simulink model "Exercitiul3"  (R2016a)
settings: Solver=VariableStepDiscrete  StartTime=0.0  StopTime=10080  RelTol=1e-3
undefined symbols (not defined in the file): m, n
settings Model: Creator=Cristina  LastModifiedBy=Cristina

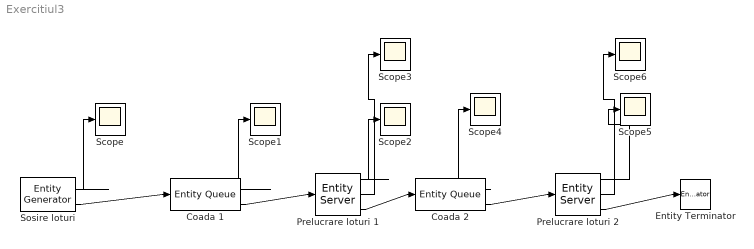
== system Exercitiul3 ==
  Coada 1 : EntityQueue  InputPortMessageModes=m  OutputPortMessageModes=n,m  Capacity=100  NumberEntitiesInBlock=on
      settings: OutputPortMap=o1,o5
  "Coada 2 " : EntityQueue  InputPortMessageModes=m  OutputPortMessageModes=n,m  Capacity=100  NumberEntitiesInBlock=on
      settings: OutputPortMap=o1,o5
  Entity Terminator : EntityTerminator  InputPortMessageModes=m
  Prelucrare loturi 1 : EntityServer  InputPortMessageModes=m  OutputPortMessageModes=n,n,m  Capacity=1  ServiceTimeValue=14  NumberEntitiesDeparted=on  Utilization=on
      settings: OutputPortMap=o0,o5,o9
  "Prelucrare loturi 2 " : EntityServer  InputPortMessageModes=m  OutputPortMessageModes=n,n,m  Capacity=1  ServiceTimeValue=3  NumberEntitiesDeparted=on  Utilization=on
      settings: OutputPortMap=o0,o5,o9
  Scope{,1..6} (7 alike) : Scope
  "Sosire loturi " : EntityGenerator  OutputPortMessageModes=n,m  TimeSource=MATLAB action  IntergenerationTimeAction=|  NumberEntitiesDeparted=on  EntityType=Structured  EntityTypeName=Entity
      | persistent init
      | if (isempty(init))
      |     rng(123);
      |     init = true;
      | end
      | dt = 12 + rand * 10;
      settings: OutputPortMap=o0,o3
  wires:
  "Sosire loturi "/2 -> Coada 1/1
  Coada 1/2 -> Prelucrare loturi 1/1
  Prelucrare loturi 1/3 -> "Coada 2 "/1
  "Coada 2 "/2 -> "Prelucrare loturi 2 "/1
  "Prelucrare loturi 2 "/3 -> Entity Terminator/1
  "Sosire loturi "/1 -> Scope/1
  Coada 1/1 -> Scope1/1
  Prelucrare loturi 1/1 -> Scope2/1
  Prelucrare loturi 1/2 -> Scope3/1
  "Coada 2 "/1 -> Scope4/1
  "Prelucrare loturi 2 "/1 -> Scope5/1
  "Prelucrare loturi 2 "/2 -> Scope6/1
